simulink model "MSICA_Projet1_StructureControle"  (R2020a)
settings: Solver=VariableStepAuto  StartTime=0.0  StopTime=10.0  RelTol=1e-3
values from neighbouring files (symbols this model uses):
  A_S1_S2 = [ zeros(3,3) eye(3) ... (first row only)    [DonneesProjet.m]
  B_S1_S2 = [zeros(3,3); inv(M_S1_S2)]    [DonneesProjet.m]
  C1 = [eye(3) zeros(3,3)]    [DonneesProjet.m]
libraries: Blocs_LTI x2
settings Model: Creator=natha  LastModifiedBy=natha
settings DebuggingCC: ArithmeticOperatorsInVariantConditions=warning
settings SFSimCC: CustomCodeUndefinedFunction=UseInterfaceOnly

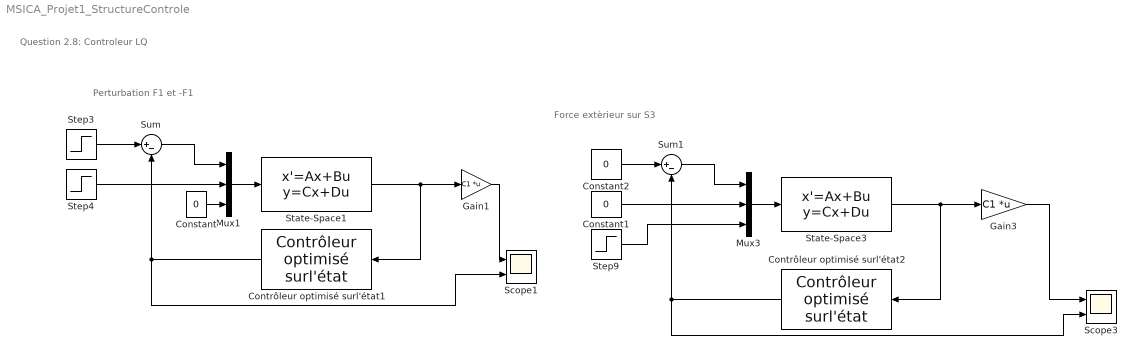
== system MSICA_Projet1_StructureControle ==
  note: Force extèrieur sur S3
  note: Perturbation F1 et -F1
  note: Question 2.8: Controleur LQ
  Constant : Constant  Value=0
  Constant1 : Constant  Value=0
  Constant2 : Constant  Value=0
  Contrôleur optimisé surl'état1 : Blocs_LTI/Contrôleur optimisé surl'état  MaskParameter1=A_S1_S2  MaskParameter2=B_S1_S2(:,1)  MaskParameter3=Q1  MaskParameter4=eye(1,1)
  Contrôleur optimisé surl'état2 : Blocs_LTI/Contrôleur optimisé surl'état  MaskParameter1=A_S1_S2  MaskParameter2=B_S1_S2(:,1)  MaskParameter3=Q2  MaskParameter4=eye(1,1)
  Gain1 : Gain  Gain=C1  Multiplication=Matrix(K*u)
  Gain3 : Gain  Gain=C1  Multiplication=Matrix(K*u)
  Mux1 : Mux  Inputs=3
  Mux3 : Mux  Inputs=3
  Scope1 : Scope  NumInputPorts=2
  Scope3 : Scope  NumInputPorts=2
  State-Space1 : StateSpace  A=A_S1_S2  B=B_S1_S2  C=eye(6)  D=zeros(6,3)  InitialCondition=0
  State-Space3 : StateSpace  A=A_S1_S2  B=B_S1_S2  C=eye(6)  D=zeros(6,3)  InitialCondition=0
  Step3 : Step  Time=0.001  Before=100  After=0  SampleTime=0
  Step4 : Step  Time=0.001  Before=-100  After=0  SampleTime=0
  Step9 : Step  Time=0.001  Before=10  After=0  SampleTime=0
  Sum : Sum  Inputs=|+-
  Sum1 : Sum  Inputs=|+-
  wires:
  Contrôleur optimisé surl'état2/1 -> Sum1/2, Scope3/2
  State-Space1/1 -> Contrôleur optimisé surl'état1/1, Gain1/1
  State-Space3/1 -> Contrôleur optimisé surl'état2/1, Gain3/1
  Gain1/1 -> Scope1/1
  Sum1/1 -> Mux3/1
  Mux3/1 -> State-Space3/1
  Sum/1 -> Mux1/1
  Step3/1 -> Sum/1
  Contrôleur optimisé surl'état1/1 -> Scope1/2, Sum/2
  Step4/1 -> Mux1/2
  Gain3/1 -> Scope3/1
  Constant1/1 -> Mux3/2
  Step9/1 -> Mux3/3
  Constant/1 -> Mux1/3
  Constant2/1 -> Sum1/1
  Mux1/1 -> State-Space1/1
